simulink model "adaptive_control_robot"  (R2016a)
settings: Solver=VariableStepAuto  StartTime=0.0  StopTime=20  RelTol=1e-3
values from neighbouring files (symbols this model uses):
  g = 9.80665    [adaptive_parameters_script.m]
  I_1 = 1.1    [adaptive_parameters_script.m]
  I_2 = 1.2    [adaptive_parameters_script.m]
  l_1 = 0.26    [adaptive_parameters_script.m]
  l_2 = 0.26    [adaptive_parameters_script.m]
  l_c1 = 0.125    [adaptive_parameters_script.m]
  l_c2 = 0.14    [adaptive_parameters_script.m]
  m_1 = 1.2    [adaptive_parameters_script.m]
  m_2 = 1.4    [adaptive_parameters_script.m]
undefined symbols (not defined in the file or in its folder): I_1_0, I_2_0, l_1_0, l_2_0, l_c1_0, l_c2_0, m_1_0, m_2_0
settings Model: Creator=USER  LastModifiedBy=dell
settings DebuggingCC: SFUnexpectedBacktrackingDiag=error  SFNoUnconditionalDefaultTransitionDiag=error
settings GRTTargetCC: TargetLangStandard=C99 (ISO)  GeneratePreprocessorConditionals=Use local settings
settings ConfigComp: CovMetricSettings=dwe  CovHtmlReporting=off  CovSaveCumulativeToWorkspaceVar=off  CovSaveSingleToWorkspaceVar=off  CovExternalEMLEnable=on

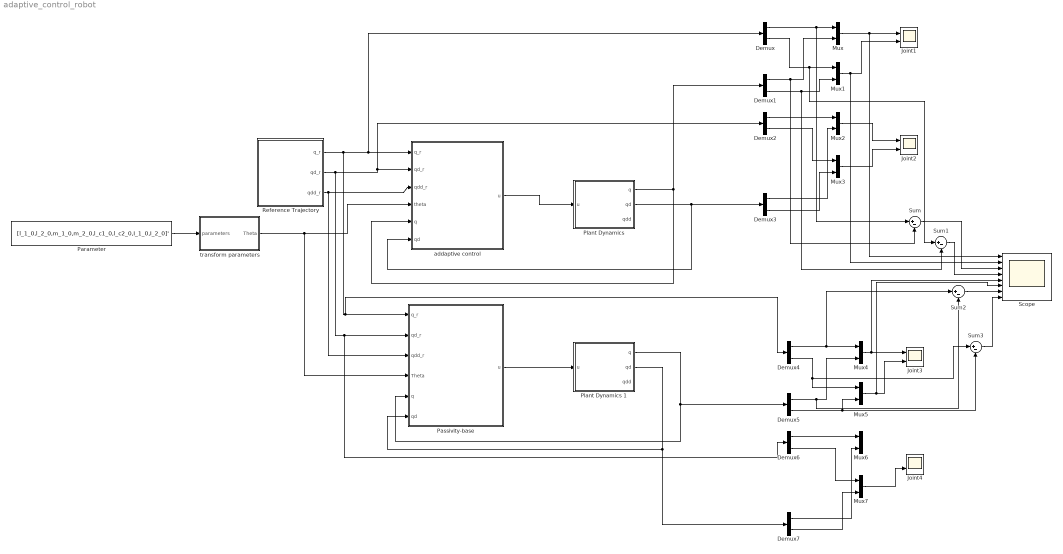
== system adaptive_control_robot ==
  Demux{,1..7} (8 alike) : Demux  Outputs=2
  Joint{1..4} (4 alike) : Scope  NumInputPorts=2
  Mux{,1..7} (8 alike) : Mux  Inputs=2
  Parameter : Constant  Value=[l_1_0,l_2_0,m_1_0,m_2_0,l_c1_0,l_c2_0,I_1_0,I_2_0]'
  Passivity-base : Subsystem  mask{lamda=diag([20 20]), K=diag([30 30])}
  "Plant Dynamics " : Subsystem
  Plant Dynamics 1 : Subsystem
  Reference Trajectory : Subsystem
  Scope : Scope  NumInputPorts=8
  Sum{,1..3} (4 alike) : Sum  Inputs=|+-
  addaptive control : Subsystem  mask{lamda=diag([10 15]), K=diag([100 100]), gamma=diag([20 15 10 20 10])}
  transform parameters : Subsystem
  wires:
  "Plant Dynamics "/2(qd) -> addaptive control/6(qd), Demux3/1
  Mux/1 -> Scope/1, Joint1/1
  Demux/1 -> Sum/1, Mux/1
  Demux1/1 -> Sum/2, Mux/2
  Mux1/1 -> Scope/2, Joint1/2
  Demux/2 -> Sum1/1, Mux1/1
  "Plant Dynamics "/1(q) -> Demux1/1, addaptive control/5(q)
  Demux1/2 -> Sum1/2, Mux1/2
  Mux2/1 -> Joint2/1
  Demux2/1 -> Mux2/1
  Demux3/1 -> Mux2/2
  Mux3/1 -> Joint2/2
  Demux2/2 -> Mux3/1
  Demux3/2 -> Mux3/2
  Parameter/1 -> transform parameters/1(parameters)
  Reference Trajectory/1(q_r) -> Demux4/1, Passivity-base/1(q_r), Demux/1, addaptive control/1(q_r)
  Reference Trajectory/2(qd_r) -> Demux6/1, Passivity-base/2(qd_r), Demux2/1, addaptive control/2(qd_r)
  Reference Trajectory/3(qdd_r) -> Passivity-base/3(qdd_r), addaptive control/3(qdd_r)
  addaptive control/1(u) -> "Plant Dynamics "/1(u)
  transform parameters/1(Theta) -> Passivity-base/4(Theta), addaptive control/4(theta)
  Passivity-base/1(u) -> Plant Dynamics 1/1(u)
  Plant Dynamics 1/1(q) -> Demux5/1, Passivity-base/5(q)
  Plant Dynamics 1/2(qd) -> Demux7/1, Passivity-base/6(qd)
  Mux4/1 -> Scope/5, Joint3/1
  Demux4/1 -> Sum2/1, Mux4/1
  Demux5/1 -> Sum2/2, Mux4/2
  Mux5/1 -> Scope/6, Joint3/2
  Demux4/2 -> Sum3/1, Mux5/1
  Demux5/2 -> Sum3/2, Mux5/2
  Demux6/1 -> Mux6/1
  Demux7/1 -> Mux6/2
  Mux7/1 -> Joint4/2
  Demux6/2 -> Mux7/1
  Demux7/2 -> Mux7/2
  Sum/1 -> Scope/3
  Sum1/1 -> Scope/4
  Sum2/1 -> Scope/7
  Sum3/1 -> Scope/8

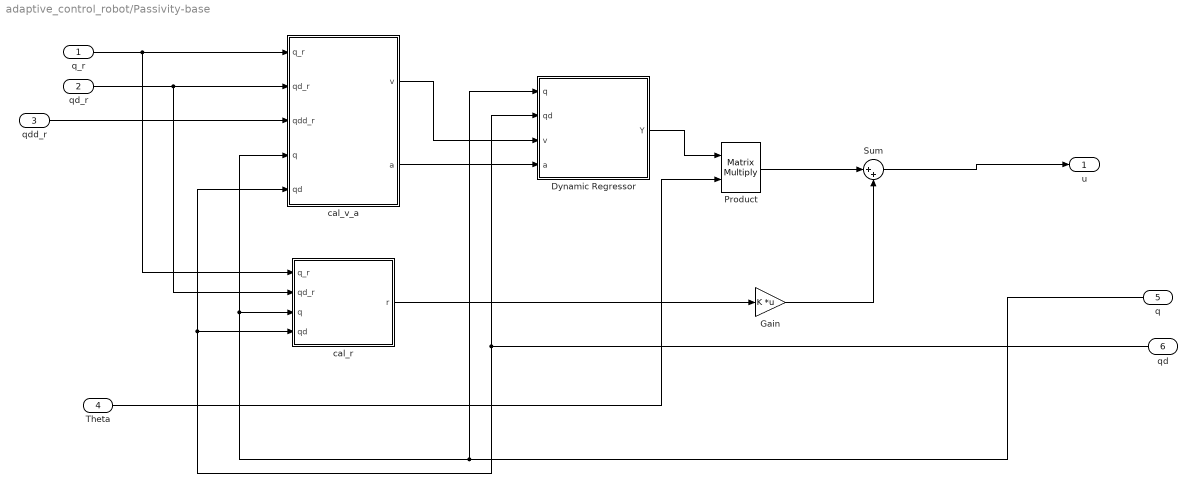
== system adaptive_control_robot/Passivity-base ==
  q_r : Inport
  qd_r : Inport  Port=2
  qdd_r : Inport  Port=3
  Theta : Inport  Port=4
  q : Inport  Port=5
  qd : Inport  Port=6
  Dynamic Regressor : Subsystem
  Gain : Gain  Gain=K  Multiplication=Matrix(K*u)
  Product : Product  Multiplication=Matrix(*)
  Sum : Sum  Inputs=|++
  cal_r : Subsystem
  cal_v_a : Subsystem
  u : Outport
  wires:
  Dynamic Regressor/1(Y) -> Product/1
  Theta/1 -> Product/2
  Product/1 -> Sum/1
  cal_v_a/2(a) -> Dynamic Regressor/4(a)
  qdd_r/1 -> cal_v_a/3(qdd_r)
  cal_r/1(r) -> Gain/1
  cal_v_a/1(v) -> Dynamic Regressor/3(v)
  Sum/1 -> u/1
  Gain/1 -> Sum/2
  q_r/1 -> cal_r/1(q_r), cal_v_a/1(q_r)
  q/1 -> Dynamic Regressor/1(q), cal_v_a/4(q), cal_r/3(q)
  qd_r/1 -> cal_r/2(qd_r), cal_v_a/2(qd_r)
  qd/1 -> Dynamic Regressor/2(qd), cal_v_a/5(qd), cal_r/4(qd)

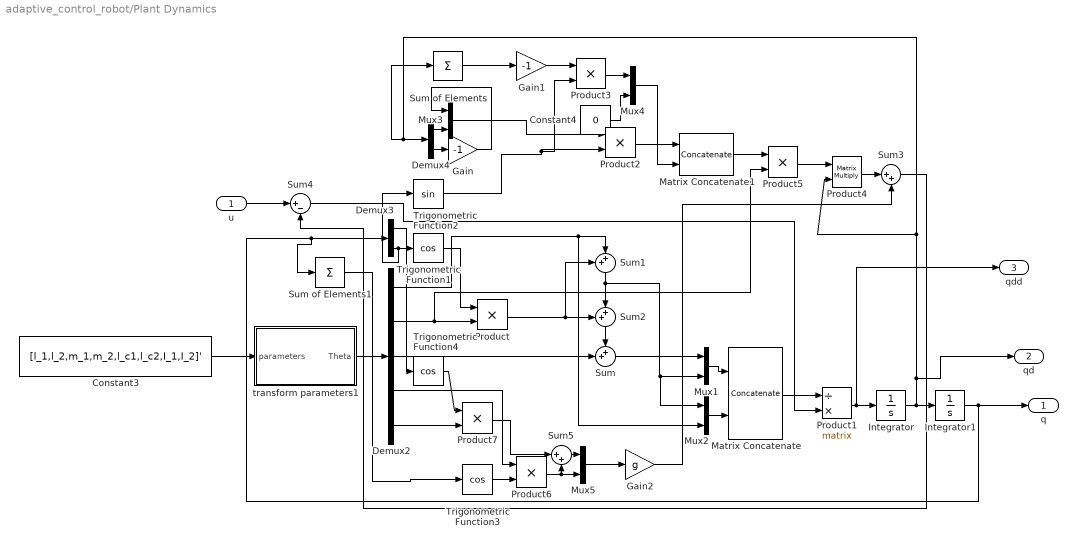
== system adaptive_control_robot/Plant Dynamics  ==
  u : Inport
  Constant3 : Constant  Value=[l_1,l_2,m_1,m_2,l_c1,l_c2,I_1,I_2]'
  Constant4 : Constant  Value=0
  Demux2 : Demux  Outputs=5
  Demux3 : Demux  Outputs=2
  Demux4 : Demux  Outputs=2
  Gain : Gain  Gain=-1
  Gain1 : Gain  Gain=-1
  Gain2 : Gain  Gain=g
  Integrator : Integrator
  Integrator1 : Integrator
  Matrix Concatenate : Concatenate  Mode=Multidimensional array  ConcatenateDimension=2
  Matrix Concatenate1 : Concatenate  Mode=Multidimensional array  ConcatenateDimension=2
  Mux{1..5} (5 alike) : Mux  Inputs=2
  Product{,2..3,5..7} (6 alike) : Product
  Product1 : Product  Inputs=/*  Multiplication=Matrix(*)
  Product4 : Product  Multiplication=Matrix(*)
  Sum : Sum  Inputs=++|
  Sum of Elements : Sum  Inputs=+
  Sum of Elements1 : Sum  Inputs=+
  Sum1 : Sum  Inputs=++|
  Sum2 : Sum  Inputs=++|
  Sum3 : Sum  Inputs=|++
  Sum4 : Sum  Inputs=|+-
  Sum5 : Sum  Inputs=|++
  Trigonometric Function1 : Trigonometry  Operator=cos
  Trigonometric Function2 : Trigonometry
  Trigonometric Function3 : Trigonometry  Operator=cos
  Trigonometric Function4 : Trigonometry  Operator=cos
  transform parameters1 : Subsystem
  q : Outport
  qd : Outport  Port=2
  qdd : Outport  Port=3
  wires:
  Product/1 -> Sum1/1, Sum2/1
  Sum1/1 -> Mux2/1, Mux1/2, Sum2/2
  Product5/1 -> Product4/1
  Gain1/1 -> Product3/1
  Trigonometric Function1/1 -> Product/1
  Sum2/1 -> Sum/1
  Trigonometric Function2/1 -> Product3/2, Product2/2
  Integrator/1 -> qd/1, Product4/2, Sum of Elements/1, Demux4/1, Integrator1/1
  Sum/1 -> Mux1/1
  Product1/1 -> qdd/1, Integrator/1
  Demux3/1 -> Trigonometric Function4/1
  Constant3/1 -> transform parameters1/1(parameters)
  Demux2/4 -> Product6/1
  Demux2/2 -> Product5/2, Product/2
  Mux1/1 -> Matrix Concatenate/1
  Product2/1 -> Matrix Concatenate1/1
  Mux2/1 -> Matrix Concatenate/2
  Sum of Elements1/1 -> Trigonometric Function3/1
  Demux2/5 -> Product7/2
  Demux4/1 -> Mux3/2
  Demux2/1 -> Mux2/2, Sum1/2
  Mux4/1 -> Matrix Concatenate1/2
  u/1 -> Sum4/1
  Sum4/1 -> Product1/2
  Integrator1/1 -> q/1, Sum of Elements1/1, Demux3/1
  Sum3/1 -> Sum4/2
  Mux3/1 -> Product2/1
  Constant4/1 -> Mux4/2
  Demux3/2 -> Trigonometric Function2/1, Trigonometric Function1/1
  Sum5/1 -> Mux5/1
  Mux5/1 -> Gain2/1
  Demux4/2 -> Gain/1
  Trigonometric Function3/1 -> Product6/2
  Demux2/3 -> Sum/2
  Matrix Concatenate/1 -> Product1/1
  Gain/1 -> Mux3/1
  Product3/1 -> Mux4/1
  Sum of Elements/1 -> Gain1/1
  Trigonometric Function4/1 -> Product7/1
  Product6/1 -> Sum5/2, Mux5/2
  Product7/1 -> Sum5/1
  Matrix Concatenate1/1 -> Product5/1
  transform parameters1/1(Theta) -> Demux2/1
  Product4/1 -> Sum3/1
  Gain2/1 -> Sum3/2

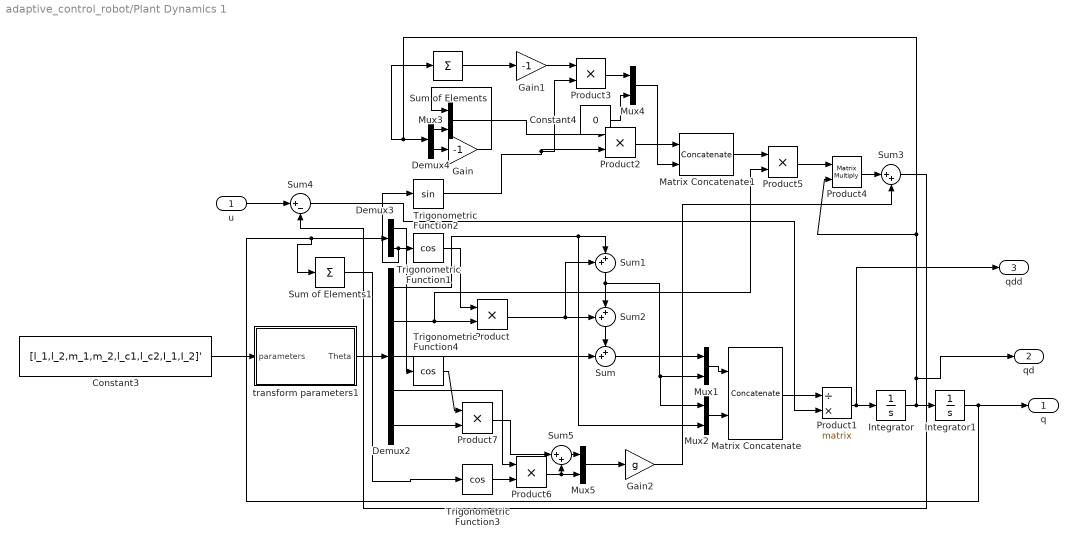
== system adaptive_control_robot/Plant Dynamics 1 ==
  u : Inport
  Constant3 : Constant  Value=[l_1,l_2,m_1,m_2,l_c1,l_c2,I_1,I_2]'
  Constant4 : Constant  Value=0
  Demux2 : Demux  Outputs=5
  Demux3 : Demux  Outputs=2
  Demux4 : Demux  Outputs=2
  Gain : Gain  Gain=-1
  Gain1 : Gain  Gain=-1
  Gain2 : Gain  Gain=g
  Integrator : Integrator
  Integrator1 : Integrator
  Matrix Concatenate : Concatenate  Mode=Multidimensional array  ConcatenateDimension=2
  Matrix Concatenate1 : Concatenate  Mode=Multidimensional array  ConcatenateDimension=2
  Mux{1..5} (5 alike) : Mux  Inputs=2
  Product{,2..3,5..7} (6 alike) : Product
  Product1 : Product  Inputs=/*  Multiplication=Matrix(*)
  Product4 : Product  Multiplication=Matrix(*)
  Sum : Sum  Inputs=++|
  Sum of Elements : Sum  Inputs=+
  Sum of Elements1 : Sum  Inputs=+
  Sum1 : Sum  Inputs=++|
  Sum2 : Sum  Inputs=++|
  Sum3 : Sum  Inputs=|++
  Sum4 : Sum  Inputs=|+-
  Sum5 : Sum  Inputs=|++
  Trigonometric Function1 : Trigonometry  Operator=cos
  Trigonometric Function2 : Trigonometry
  Trigonometric Function3 : Trigonometry  Operator=cos
  Trigonometric Function4 : Trigonometry  Operator=cos
  transform parameters1 : Subsystem
  q : Outport
  qd : Outport  Port=2
  qdd : Outport  Port=3
  wires:
  Gain2/1 -> Sum3/2
  Product4/1 -> Sum3/1
  transform parameters1/1(Theta) -> Demux2/1
  Matrix Concatenate1/1 -> Product5/1
  Product7/1 -> Sum5/1
  Product6/1 -> Mux5/2, Sum5/2
  Trigonometric Function4/1 -> Product7/1
  Sum of Elements/1 -> Gain1/1
  Product3/1 -> Mux4/1
  Gain/1 -> Mux3/1
  Matrix Concatenate/1 -> Product1/1
  Demux2/3 -> Sum/2
  Trigonometric Function3/1 -> Product6/2
  Demux4/2 -> Gain/1
  Mux5/1 -> Gain2/1
  Sum5/1 -> Mux5/1
  Demux3/2 -> Trigonometric Function1/1, Trigonometric Function2/1
  Constant4/1 -> Mux4/2
  Mux3/1 -> Product2/1
  Sum3/1 -> Sum4/2
  Integrator1/1 -> Demux3/1, Sum of Elements1/1, q/1
  Sum4/1 -> Product1/2
  u/1 -> Sum4/1
  Mux4/1 -> Matrix Concatenate1/2
  Demux2/1 -> Sum1/2, Mux2/2
  Demux4/1 -> Mux3/2
  Demux2/5 -> Product7/2
  Sum of Elements1/1 -> Trigonometric Function3/1
  Mux2/1 -> Matrix Concatenate/2
  Product2/1 -> Matrix Concatenate1/1
  Mux1/1 -> Matrix Concatenate/1
  Demux2/2 -> Product/2, Product5/2
  Demux2/4 -> Product6/1
  Constant3/1 -> transform parameters1/1(parameters)
  Demux3/1 -> Trigonometric Function4/1
  Product1/1 -> Integrator/1, qdd/1
  Sum/1 -> Mux1/1
  Integrator/1 -> Integrator1/1, Demux4/1, Sum of Elements/1, Product4/2, qd/1
  Trigonometric Function2/1 -> Product2/2, Product3/2
  Sum2/1 -> Sum/1
  Trigonometric Function1/1 -> Product/1
  Gain1/1 -> Product3/1
  Product5/1 -> Product4/1
  Sum1/1 -> Sum2/2, Mux1/2, Mux2/1
  Product/1 -> Sum2/1, Sum1/1

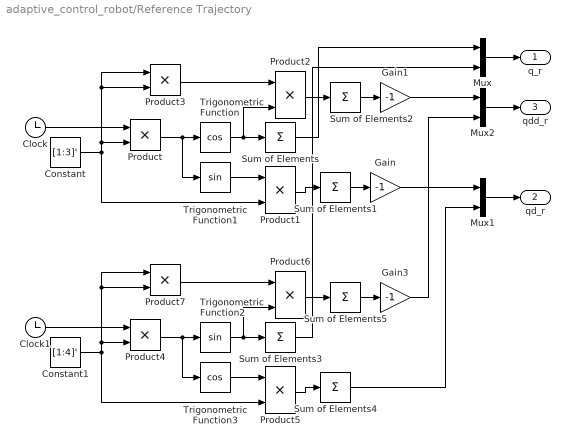
== system adaptive_control_robot/Reference Trajectory ==
  Clock : Clock
  Clock1 : Clock
  Constant : Constant  Value=[1:3]'
  Constant1 : Constant  Value=[1:4]'
  Gain : Gain  Gain=-1
  Gain1 : Gain  Gain=-1
  Gain3 : Gain  Gain=-1
  Mux : Mux  Inputs=2
  Mux1 : Mux  Inputs=2
  Mux2 : Mux  Inputs=2
  Product{,1..7} (8 alike) : Product
  Sum of Elements{,1..5} (6 alike) : Sum  Inputs=+
  Trigonometric Function : Trigonometry  Operator=cos
  Trigonometric Function1 : Trigonometry
  Trigonometric Function2 : Trigonometry
  Trigonometric Function3 : Trigonometry  Operator=cos
  q_r : Outport
  qd_r : Outport  Port=2
  qdd_r : Outport  Port=3
  wires:
  Sum of Elements1/1 -> Gain/1
  Sum of Elements3/1 -> Mux/2
  Gain3/1 -> Mux2/2
  Constant/1 -> Product1/2, Product/2, Product3/1, Product3/2
  Product1/1 -> Sum of Elements1/1
  Sum of Elements/1 -> Mux/1
  Trigonometric Function1/1 -> Product1/1
  Sum of Elements4/1 -> Mux1/2
  Product2/1 -> Sum of Elements2/1
  Product3/1 -> Product2/1
  Gain1/1 -> Mux2/1
  Sum of Elements2/1 -> Gain1/1
  Product5/1 -> Sum of Elements4/1
  Trigonometric Function2/1 -> Product6/2, Sum of Elements3/1
  Clock1/1 -> Product4/1
  Sum of Elements5/1 -> Gain3/1
  Product7/1 -> Product6/1
  Constant1/1 -> Product5/2, Product4/2, Product7/1, Product7/2
  Trigonometric Function3/1 -> Product5/1
  Product6/1 -> Sum of Elements5/1
  Product4/1 -> Trigonometric Function3/1, Trigonometric Function2/1
  Mux/1 -> q_r/1
  Mux1/1 -> qd_r/1
  Mux2/1 -> qdd_r/1
  Product/1 -> Trigonometric Function1/1, Trigonometric Function/1
  Clock/1 -> Product/1
  Trigonometric Function/1 -> Product2/2, Sum of Elements/1
  Gain/1 -> Mux1/1

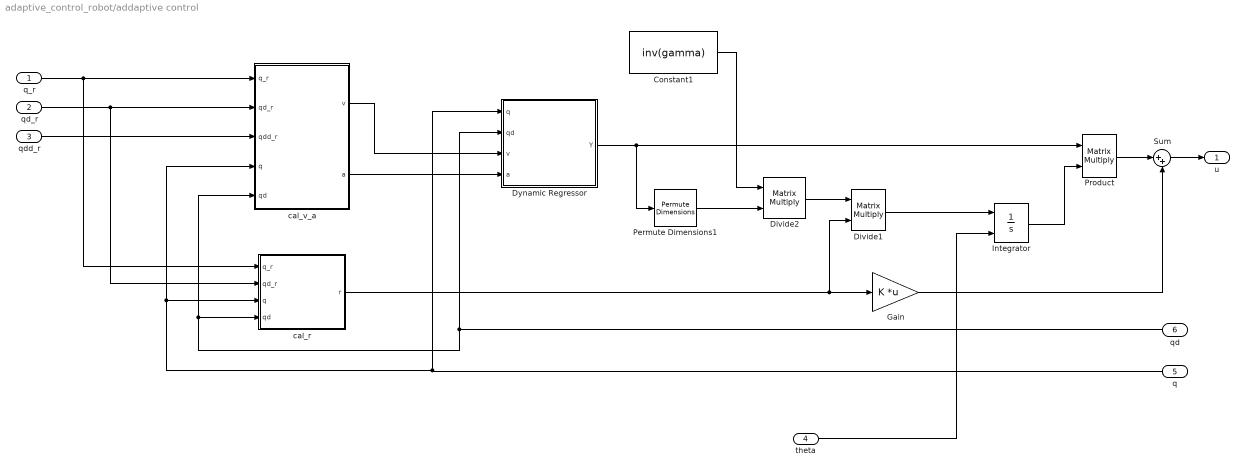
== system adaptive_control_robot/addaptive control ==
  q_r : Inport
  qd_r : Inport  Port=2
  qdd_r : Inport  Port=3
  theta : Inport  Port=4
  q : Inport  Port=5
  qd : Inport  Port=6
  Constant1 : Constant  Value=inv(gamma)
  Divide1 : Product  Inputs=**  Multiplication=Matrix(*)
  Divide2 : Product  Inputs=**  Multiplication=Matrix(*)
  Dynamic Regressor : Subsystem
  Gain : Gain  Gain=K  Multiplication=Matrix(K*u)
  Integrator : Integrator  InitialConditionSource=external
  Permute Dimensions1 : PermuteDimensions
  Product : Product  Multiplication=Matrix(*)
  Sum : Sum  Inputs=|++
  cal_r : Subsystem
  cal_v_a : Subsystem
  u : Outport
  wires:
  qd_r/1 -> cal_v_a/2(qd_r), cal_r/2(qd_r)
  q_r/1 -> cal_v_a/1(q_r), cal_r/1(q_r)
  Gain/1 -> Sum/2
  Sum/1 -> u/1
  qdd_r/1 -> cal_v_a/3(qdd_r)
  Product/1 -> Sum/1
  Dynamic Regressor/1(Y) -> Permute Dimensions1/1, Product/1
  cal_r/1(r) -> Divide1/2, Gain/1
  qd/1 -> cal_v_a/5(qd), cal_r/4(qd), Dynamic Regressor/2(qd)
  q/1 -> Dynamic Regressor/1(q), cal_r/3(q), cal_v_a/4(q)
  cal_v_a/1(v) -> Dynamic Regressor/3(v)
  cal_v_a/2(a) -> Dynamic Regressor/4(a)
  Constant1/1 -> Divide2/1
  Integrator/1 -> Product/2
  Permute Dimensions1/1 -> Divide2/2
  theta/1 -> Integrator/2
  Divide2/1 -> Divide1/1
  Divide1/1 -> Integrator/1

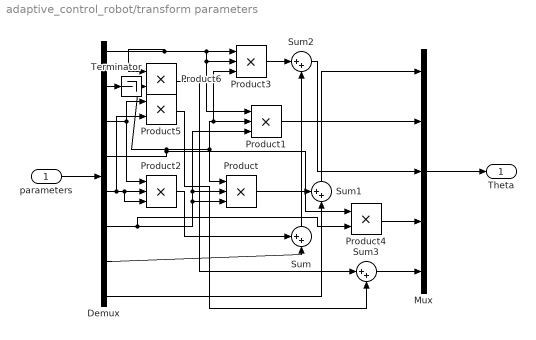
== system adaptive_control_robot/transform parameters ==
  parameters : Inport
  Demux : Demux  Outputs=8
  Mux : Mux  Inputs=5
  Product{,1..3} (4 alike) : Product  Inputs=3
  Product4 : Product
  Product5 : Product
  Product6 : Product
  Sum : Sum  Inputs=++|
  Sum1 : Sum  Inputs=++|
  Sum2 : Sum  Inputs=|++
  Sum3 : Sum  Inputs=|++
  Terminator : Terminator
  Theta : Outport
  wires:
  Sum3/1 -> Mux/5
  Product5/1 -> Sum3/2
  Product3/1 -> Sum2/1
  Mux/1 -> Theta/1
  Sum2/1 -> Mux/3
  Demux/2 -> Terminator/1
  Product6/1 -> Sum3/1
  Sum/1 -> Sum2/2
  Demux/3 -> Product5/1, Product2/1
  Demux/1 -> Product6/1, Product3/1, Product3/2, Product1/1
  Product1/1 -> Mux/2
  parameters/1 -> Demux/1
  Demux/4 -> Product4/1, Product3/3, Product1/2, Product/1, Product6/2
  Demux/5 -> Product5/2, Product2/3, Product2/2
  Demux/6 -> Product4/2, Product1/3, Product/2, Product/3
  Product4/1 -> Mux/4
  Sum1/1 -> Mux/1
  Product/1 -> Sum1/1
  Demux/7 -> Sum/2
  Demux/8 -> Sum1/2
  Product2/1 -> Sum/1

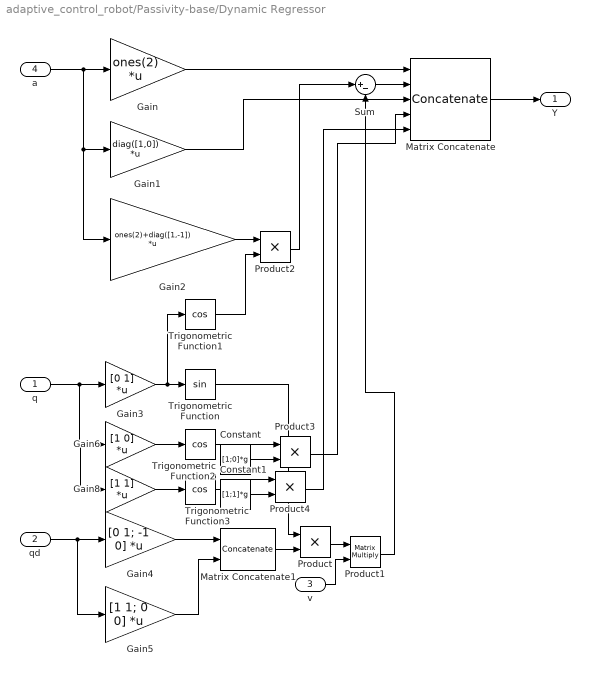
== system adaptive_control_robot/Passivity-base/Dynamic Regressor ==
  q : Inport
  qd : Inport  Port=2
  v : Inport  Port=3
  a : Inport  Port=4
  Constant : Constant  Value=[1;0]*g
  Constant1 : Constant  Value=[1;1]*g
  Gain : Gain  Gain=ones(2)  Multiplication=Matrix(K*u)
  Gain1 : Gain  Gain=diag([1,0])  Multiplication=Matrix(K*u)
  Gain2 : Gain  Gain=ones(2)+diag([1,-1])  Multiplication=Matrix(K*u)
  Gain3 : Gain  Gain=[0 1]  Multiplication=Matrix(K*u)
  Gain4 : Gain  Gain=[0 1; -1 0]  Multiplication=Matrix(K*u)
  Gain5 : Gain  Gain=[1 1; 0 0]  Multiplication=Matrix(K*u)
  Gain6 : Gain  Gain=[1 0]  Multiplication=Matrix(K*u)
  Gain8 : Gain  Gain=[1 1]  Multiplication=Matrix(K*u)
  Matrix Concatenate : Concatenate  NumInputs=5  Mode=Multidimensional array  ConcatenateDimension=2
  Matrix Concatenate1 : Concatenate  Mode=Multidimensional array  ConcatenateDimension=2
  Product{,2..4} (4 alike) : Product
  Product1 : Product  Multiplication=Matrix(*)
  Sum : Sum  Inputs=|+-
  Trigonometric Function : Trigonometry
  Trigonometric Function1 : Trigonometry  Operator=cos
  Trigonometric Function2 : Trigonometry  Operator=cos
  Trigonometric Function3 : Trigonometry  Operator=cos
  Y : Outport
  wires:
  Product2/1 -> Sum/1
  a/1 -> Gain2/1, Gain1/1, Gain/1
  qd/1 -> Gain5/1, Gain4/1
  Matrix Concatenate1/1 -> Product/2
  Gain3/1 -> Trigonometric Function1/1, Trigonometric Function/1
  Gain1/1 -> Matrix Concatenate/3
  Gain5/1 -> Matrix Concatenate1/2
  Trigonometric Function/1 -> Product/1
  Gain/1 -> Matrix Concatenate/1
  Gain4/1 -> Matrix Concatenate1/1
  q/1 -> Gain8/1, Gain6/1, Gain3/1
  Product1/1 -> Sum/2
  Product/1 -> Product1/1
  Sum/1 -> Matrix Concatenate/2
  v/1 -> Product1/2
  Gain6/1 -> Trigonometric Function2/1
  Trigonometric Function3/1 -> Product4/1
  Gain8/1 -> Trigonometric Function3/1
  Trigonometric Function2/1 -> Product3/1
  Matrix Concatenate/1 -> Y/1
  Product4/1 -> Matrix Concatenate/4
  Trigonometric Function1/1 -> Product2/2
  Product3/1 -> Matrix Concatenate/5
  Gain2/1 -> Product2/1
  Constant/1 -> Product3/2
  Constant1/1 -> Product4/2

== system adaptive_control_robot/Passivity-base/cal_r ==
  q_r : Inport
  qd_r : Inport  Port=2
  q : Inport  Port=3
  qd : Inport  Port=4
  Subtract : Sum  Inputs=+-
  Subtract1 : Sum  Inputs=+-
  Sum1 : Sum  Inputs=|++
  lamda : Gain  Gain=lamda  Multiplication=Matrix(K*u)
  r : Outport
  wires:
  qd_r/1 -> Subtract/1
  qd/1 -> Subtract/2
  q_r/1 -> Subtract1/1
  lamda/1 -> Sum1/1
  q/1 -> Subtract1/2
  Sum1/1 -> r/1
  Subtract1/1 -> lamda/1
  Subtract/1 -> Sum1/2

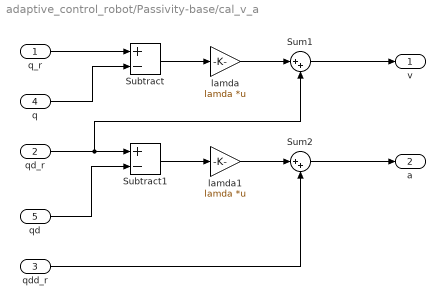
== system adaptive_control_robot/Passivity-base/cal_v_a ==
  q_r : Inport
  qd_r : Inport  Port=2
  qdd_r : Inport  Port=3
  q : Inport  Port=4
  qd : Inport  Port=5
  Subtract : Sum  Inputs=+-
  Subtract1 : Sum  Inputs=+-
  Sum1 : Sum  Inputs=|++
  Sum2 : Sum  Inputs=|++
  lamda : Gain  Gain=lamda  Multiplication=Matrix(K*u)
  lamda1 : Gain  Gain=lamda  Multiplication=Matrix(K*u)
  v : Outport
  a : Outport  Port=2
  wires:
  lamda/1 -> Sum1/1
  Sum1/1 -> v/1
  Sum2/1 -> a/1
  qdd_r/1 -> Sum2/2
  lamda1/1 -> Sum2/1
  q_r/1 -> Subtract/1
  qd/1 -> Subtract1/2
  qd_r/1 -> Sum1/2, Subtract1/1
  Subtract1/1 -> lamda1/1
  Subtract/1 -> lamda/1
  q/1 -> Subtract/2

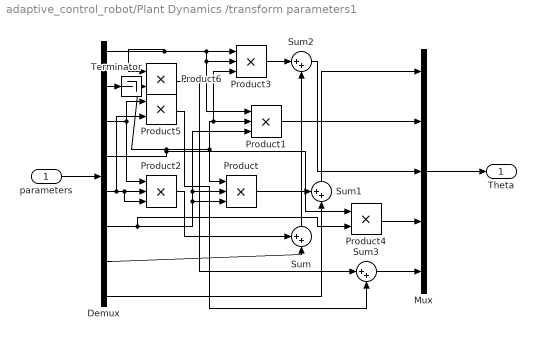
== system adaptive_control_robot/Plant Dynamics /transform parameters1 ==
  parameters : Inport
  Demux : Demux  Outputs=8
  Mux : Mux  Inputs=5
  Product{,1..3} (4 alike) : Product  Inputs=3
  Product4 : Product
  Product5 : Product
  Product6 : Product
  Sum : Sum  Inputs=++|
  Sum1 : Sum  Inputs=++|
  Sum2 : Sum  Inputs=|++
  Sum3 : Sum  Inputs=|++
  Terminator : Terminator
  Theta : Outport
  wires:
  Sum3/1 -> Mux/5
  Product5/1 -> Sum3/2
  Product3/1 -> Sum2/1
  Mux/1 -> Theta/1
  Sum2/1 -> Mux/3
  Demux/2 -> Terminator/1
  Product6/1 -> Sum3/1
  Sum/1 -> Sum2/2
  Demux/3 -> Product5/1, Product2/1
  Demux/1 -> Product6/1, Product3/1, Product3/2, Product1/1
  Product1/1 -> Mux/2
  parameters/1 -> Demux/1
  Demux/4 -> Product4/1, Product3/3, Product1/2, Product/1, Product6/2
  Demux/5 -> Product5/2, Product2/3, Product2/2
  Demux/6 -> Product4/2, Product1/3, Product/2, Product/3
  Product4/1 -> Mux/4
  Sum1/1 -> Mux/1
  Product/1 -> Sum1/1
  Demux/7 -> Sum/2
  Demux/8 -> Sum1/2
  Product2/1 -> Sum/1

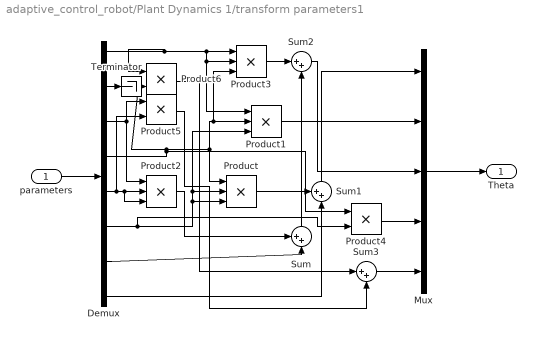
== system adaptive_control_robot/Plant Dynamics 1/transform parameters1 ==
  parameters : Inport
  Demux : Demux  Outputs=8
  Mux : Mux  Inputs=5
  Product{,1..3} (4 alike) : Product  Inputs=3
  Product4 : Product
  Product5 : Product
  Product6 : Product
  Sum : Sum  Inputs=++|
  Sum1 : Sum  Inputs=++|
  Sum2 : Sum  Inputs=|++
  Sum3 : Sum  Inputs=|++
  Terminator : Terminator
  Theta : Outport
  wires:
  Product2/1 -> Sum/1
  Demux/8 -> Sum1/2
  Demux/7 -> Sum/2
  Product/1 -> Sum1/1
  Sum1/1 -> Mux/1
  Product4/1 -> Mux/4
  Demux/6 -> Product/3, Product/2, Product1/3, Product4/2
  Demux/5 -> Product2/2, Product2/3, Product5/2
  Demux/4 -> Product6/2, Product/1, Product1/2, Product3/3, Product4/1
  parameters/1 -> Demux/1
  Product1/1 -> Mux/2
  Demux/1 -> Product1/1, Product3/2, Product3/1, Product6/1
  Demux/3 -> Product2/1, Product5/1
  Sum/1 -> Sum2/2
  Product6/1 -> Sum3/1
  Demux/2 -> Terminator/1
  Sum2/1 -> Mux/3
  Mux/1 -> Theta/1
  Product3/1 -> Sum2/1
  Product5/1 -> Sum3/2
  Sum3/1 -> Mux/5

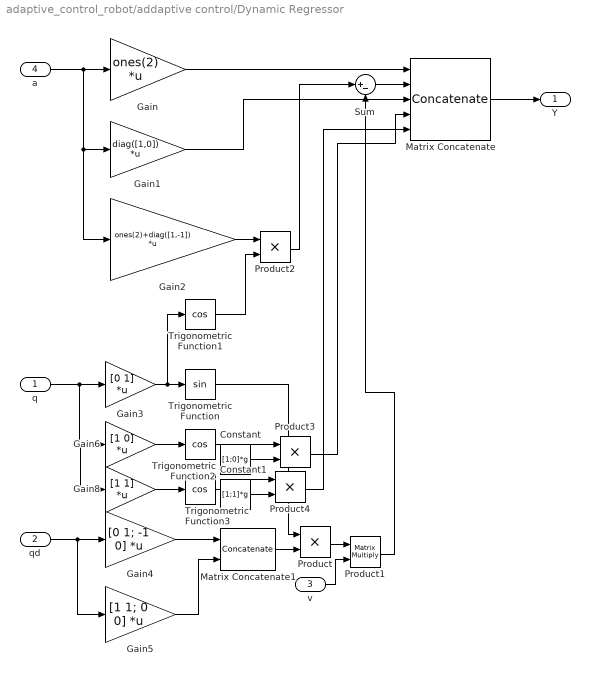
== system adaptive_control_robot/addaptive control/Dynamic Regressor ==
  q : Inport
  qd : Inport  Port=2
  v : Inport  Port=3
  a : Inport  Port=4
  Constant : Constant  Value=[1;0]*g
  Constant1 : Constant  Value=[1;1]*g
  Gain : Gain  Gain=ones(2)  Multiplication=Matrix(K*u)
  Gain1 : Gain  Gain=diag([1,0])  Multiplication=Matrix(K*u)
  Gain2 : Gain  Gain=ones(2)+diag([1,-1])  Multiplication=Matrix(K*u)
  Gain3 : Gain  Gain=[0 1]  Multiplication=Matrix(K*u)
  Gain4 : Gain  Gain=[0 1; -1 0]  Multiplication=Matrix(K*u)
  Gain5 : Gain  Gain=[1 1; 0 0]  Multiplication=Matrix(K*u)
  Gain6 : Gain  Gain=[1 0]  Multiplication=Matrix(K*u)
  Gain8 : Gain  Gain=[1 1]  Multiplication=Matrix(K*u)
  Matrix Concatenate : Concatenate  NumInputs=5  Mode=Multidimensional array  ConcatenateDimension=2
  Matrix Concatenate1 : Concatenate  Mode=Multidimensional array  ConcatenateDimension=2
  Product{,2..4} (4 alike) : Product
  Product1 : Product  Multiplication=Matrix(*)
  Sum : Sum  Inputs=|+-
  Trigonometric Function : Trigonometry
  Trigonometric Function1 : Trigonometry  Operator=cos
  Trigonometric Function2 : Trigonometry  Operator=cos
  Trigonometric Function3 : Trigonometry  Operator=cos
  Y : Outport
  wires:
  Constant1/1 -> Product4/2
  Constant/1 -> Product3/2
  Gain2/1 -> Product2/1
  Product3/1 -> Matrix Concatenate/5
  Trigonometric Function1/1 -> Product2/2
  Product4/1 -> Matrix Concatenate/4
  Matrix Concatenate/1 -> Y/1
  Trigonometric Function2/1 -> Product3/1
  Gain8/1 -> Trigonometric Function3/1
  Trigonometric Function3/1 -> Product4/1
  Gain6/1 -> Trigonometric Function2/1
  v/1 -> Product1/2
  Sum/1 -> Matrix Concatenate/2
  Product/1 -> Product1/1
  Product1/1 -> Sum/2
  q/1 -> Gain3/1, Gain6/1, Gain8/1
  Gain4/1 -> Matrix Concatenate1/1
  Gain/1 -> Matrix Concatenate/1
  Trigonometric Function/1 -> Product/1
  Gain5/1 -> Matrix Concatenate1/2
  Gain1/1 -> Matrix Concatenate/3
  Gain3/1 -> Trigonometric Function/1, Trigonometric Function1/1
  Matrix Concatenate1/1 -> Product/2
  qd/1 -> Gain4/1, Gain5/1
  a/1 -> Gain/1, Gain1/1, Gain2/1
  Product2/1 -> Sum/1

== system adaptive_control_robot/addaptive control/cal_r ==
  q_r : Inport
  qd_r : Inport  Port=2
  q : Inport  Port=3
  qd : Inport  Port=4
  Subtract : Sum  Inputs=+-
  Subtract1 : Sum  Inputs=+-
  Sum1 : Sum  Inputs=|++
  lamda : Gain  Gain=lamda  Multiplication=Matrix(K*u)
  r : Outport
  wires:
  Subtract/1 -> Sum1/2
  Subtract1/1 -> lamda/1
  Sum1/1 -> r/1
  q/1 -> Subtract1/2
  lamda/1 -> Sum1/1
  q_r/1 -> Subtract1/1
  qd/1 -> Subtract/2
  qd_r/1 -> Subtract/1

== system adaptive_control_robot/addaptive control/cal_v_a ==
  q_r : Inport
  qd_r : Inport  Port=2
  qdd_r : Inport  Port=3
  q : Inport  Port=4
  qd : Inport  Port=5
  Subtract : Sum  Inputs=+-
  Subtract1 : Sum  Inputs=+-
  Sum1 : Sum  Inputs=|++
  Sum2 : Sum  Inputs=|++
  lamda : Gain  Gain=lamda  Multiplication=Matrix(K*u)
  lamda1 : Gain  Gain=lamda  Multiplication=Matrix(K*u)
  v : Outport
  a : Outport  Port=2
  wires:
  q/1 -> Subtract/2
  Subtract/1 -> lamda/1
  Subtract1/1 -> lamda1/1
  qd_r/1 -> Subtract1/1, Sum1/2
  qd/1 -> Subtract1/2
  q_r/1 -> Subtract/1
  lamda1/1 -> Sum2/1
  qdd_r/1 -> Sum2/2
  Sum2/1 -> a/1
  Sum1/1 -> v/1
  lamda/1 -> Sum1/1
